simulink library "BMS_plant_lib"  (R2022b)
settings: Solver=VariableStepAuto  StartTime=0.0  StopTime=10.0  RelTol=1e-3
settings Model: Creator=LinF  LastModifiedBy=LinF

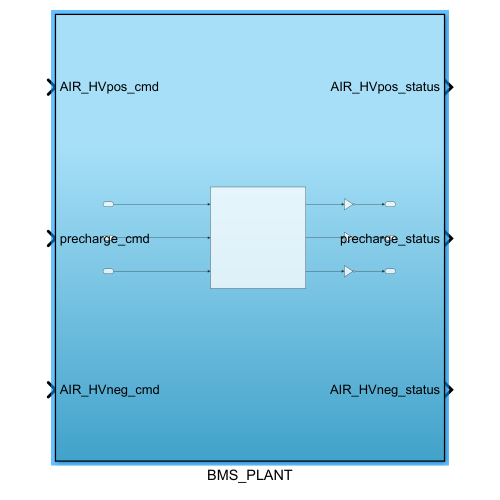
[thumbnail: Simulink's stored preview of the top-level diagram]
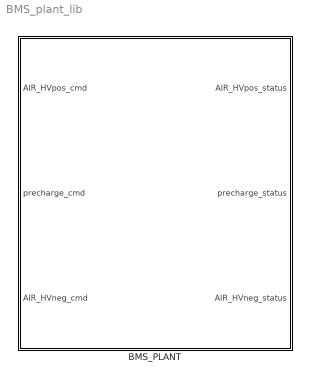
== system BMS_plant_lib ==
  BMS_PLANT : Subsystem

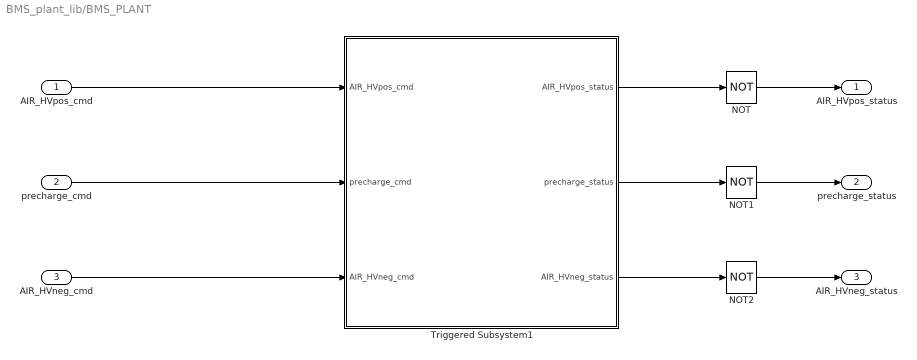
== system BMS_plant_lib/BMS_PLANT ==
  AIR_HVpos_cmd : Inport
  precharge_cmd : Inport  Port=2
  AIR_HVneg_cmd : Inport  Port=3
  NOT : Logic  Operator=NOT  IconShape=distinctive  AllPortsSameDT=off  OutDataTypeStr=boolean
  NOT1 : Logic  Operator=NOT  IconShape=distinctive  AllPortsSameDT=off  OutDataTypeStr=boolean
  NOT2 : Logic  Operator=NOT  IconShape=distinctive  AllPortsSameDT=off  OutDataTypeStr=boolean
  Triggered Subsystem1 : Subsystem  TreatAsAtomicUnit=on
  AIR_HVpos_status : Outport
  precharge_status : Outport  Port=2
  AIR_HVneg_status : Outport  Port=3
  wires:
  AIR_HVpos_cmd/1 -> Triggered Subsystem1/1(AIR_HVpos_cmd)
  precharge_cmd/1 -> Triggered Subsystem1/2(precharge_cmd)
  AIR_HVneg_cmd/1 -> Triggered Subsystem1/3(AIR_HVneg_cmd)
  Triggered Subsystem1/1(AIR_HVpos_status) -> NOT/1
  Triggered Subsystem1/2(precharge_status) -> NOT1/1
  Triggered Subsystem1/3(AIR_HVneg_status) -> NOT2/1
  NOT/1 -> AIR_HVpos_status/1
  NOT1/1 -> precharge_status/1
  NOT2/1 -> AIR_HVneg_status/1

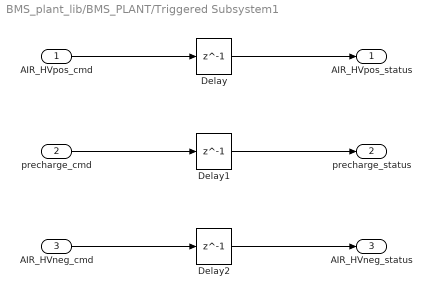
== system BMS_plant_lib/BMS_PLANT/Triggered Subsystem1 ==
  AIR_HVpos_cmd : Inport
  precharge_cmd : Inport  Port=2
  AIR_HVneg_cmd : Inport  Port=3
  Delay : Delay  DelayLength=1
  Delay1 : Delay  DelayLength=1
  Delay2 : Delay  DelayLength=1
  AIR_HVpos_status : Outport
  precharge_status : Outport  Port=2
  AIR_HVneg_status : Outport  Port=3
  wires:
  AIR_HVneg_cmd/1 -> Delay2/1
  precharge_cmd/1 -> Delay1/1
  Delay/1 -> AIR_HVpos_status/1
  AIR_HVpos_cmd/1 -> Delay/1
  Delay1/1 -> precharge_status/1
  Delay2/1 -> AIR_HVneg_status/1
